simulink model "LM_dyn"  (Simulink 7.9)
settings: Solver=ode4  StartTime=0.0  StopTime=tmax-1  FixedStep=dt  RelTol=1e-3
values from neighbouring files (symbols this model uses):
  dt = 1    [ISLM1.m]    (also in ISLM2.m)
  model_str = regexprep(model_str,'\/','\.\/')    [ISLM1.m]    (also in ISLM2.m)
settings Model: Creator=danai  LastModifiedBy=Kourosh Danai
settings SolverCC: MaxConsecutiveMinStep=dt

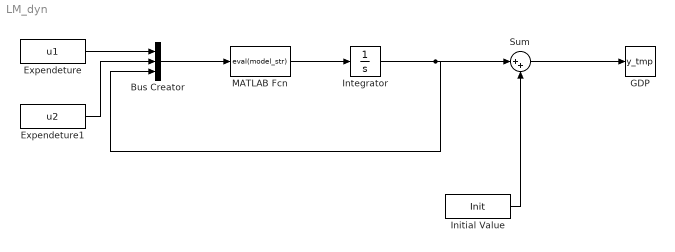
== system LM_dyn ==
  Bus Creator : BusCreator  Inputs=3
  Expendeture : FromWorkspace  VariableName=u1  OutDataTypeStr=double  SampleTime=dt
  Expendeture1 : FromWorkspace  VariableName=u2  OutDataTypeStr=double  SampleTime=dt
  GDP : ToWorkspace  VariableName=y_tmp  SampleTime=-1
  Initial Value : FromWorkspace  VariableName=Init  OutDataTypeStr=double  SampleTime=dt
  Integrator : Integrator
  MATLAB Fcn : MATLABFcn  MATLABFcn=eval(model_str)
  Sum : Sum  Inputs=|++
  wires:
  Expendeture/1 -> Bus Creator/1
  Bus Creator/1 -> MATLAB Fcn/1
  MATLAB Fcn/1 -> Integrator/1
  Integrator/1 -> Sum/1, Bus Creator/3
  Initial Value/1 -> Sum/2
  Sum/1 -> GDP/1
  Expendeture1/1 -> Bus Creator/2
